simulink model "quantis_filter_1"  (Simulink 7.8)
settings: Solver=FixedStepDiscrete  StartTime=0.0  StopTime=1  RelTol=1e-3
values from neighbouring files (symbols this model uses):
  fs = 16000    [G722_1.m]    (also in TP_fdesign1.m = 0.215; adaptiv_2.m = 1000; adaptiv_3.m = 1000; adaptiv_4.m = 1000)
undefined symbols (not defined in the file or in its folder): dfilt, frs
libraries: dsparch4 x1, dspsrcs4 x1
settings Model: Creator=svenhoffmann  LastModifiedBy=josef  ExtModeAutoUpdateStatusClock=off
settings OptimizationCC: InlineInvariantSignals=on  InitFltsAndDblsToZero=on
settings DebuggingCC: SaveWithParameterizedLinksMsg=none  SignalResolutionControl=TryResolveAllWithWarning  MultiTaskDSMMsg=warning  MultiTaskCondExecSysMsg=none  FcnCallInpInsideContextMsg=Use local settings  StrictBusMsg=None
settings RTWCC: IncludeERTFirstTime=on
settings GRTTargetCC: TargetFcnLib=ansi_tfl_tmw.mat

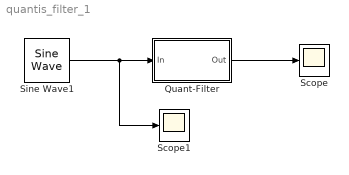
== system quantis_filter_1 ==
  Quant-Filter : Subsystem  Tag=BlockMethodSubSystem
  Scope : Scope
  Scope1 : Scope
  Sine Wave1 : dspsrcs4/Sine Wave  Amplitude=0.95  Frequency=fs/round(1/frs)  Phase=0  SampleMode=Discrete  OutComplex=Real  CompMethod=Table lookup  TableSize=Speed  SampleTime=1/fs  SamplesPerFrame=1  ResetState=Restart at time zero  dataType=User-defined  wordLen=16  udDataType=sfix(16)  fracBitsMode=User-defined  numFracBits=15  OutDataTypeStr=fixdt(1,16)  LastOutDataTypeStr=fixdt(1,16)
  wires:
  Sine Wave1/1 -> Quant-Filter/1(In), Scope1/1
  Quant-Filter/1(Out) -> Scope/1

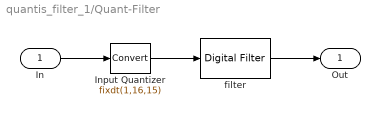
== system quantis_filter_1/Quant-Filter ==
  In : Inport
  Input Quantizer : DataTypeConversion  OutDataTypeStr=fixdt(1,16,15)  RndMeth=Round  SaturateOnIntegerOverflow=on
  filter : dsparch4/Digital Filter  TypePopup=IIR (poles & zeros)  IIRFiltStruct=Direct form II  AllPoleFiltStruct=Direct form  FIRFiltStruct=Direct form  CoeffSource=Specify via dialog  NumCoeffs=[0.000288582897651351 -0.00033839318745116 -0.000390339936011391 -0.000259639046498942 7.38443078093614e-05 0.000357868370809173 0.000300939938371918 -0.000105129054930465 -0.00050182175147418 -0.000461335623672789 7.11317455494947e-05 0.000639924106940051 0.000655538279003823 -8.41836808940086e-06 -0.000791306426059373 -0.000901062859792003 -0.000100245580998996 0.000946038863637751 0.00120070496164748 0.000266513423161963 -0.00109528806843289 -0.00155788027039267 -0.000504175926187551 0.0012271638548347 0.00197432303656502 0.000828029512424704 -0.00132731841121327 -0.00245007010985775 -0.00125334653945962 0.00137873110724473 0.00298262555164426 0.00179638152844382 -0.00136038330873108 -0.00356731415934766 -0.0024752313224474 0.00124855058800306 0.00419864437922346 0.00330857950612985 -0.00101484760130196 -0.00486584907866968 -0.00431926877262247 0.000626112664150373 0.00555922195206759 0.00553337686591329 -4.06558700779738e-05 -0.00626541757131323 -0.00698518729854155 -0.000793203461600921 0.0069706742258114 0.00872392161471349 0.00194621229973601 -0.00765928347665411 -0.0108228080449625 -0.00351974772730628 0.00831542716470059 0.013400989063819 0.00567168379746354 -0.00892343070006198 -0.0166661145296759 -0.00867205472801053 0.00946779586510596 0.0210119633125462 0.0130342493783314 -0.0099347473329221 -0.0272758084634068 -0.0198850138076668 0.0103117218369764 0.0375727529685634 0.0322854051395793 -0.0105884468313137 -0.0591349841236665 -0.0624946230301509 0.0107577655260804 0.142692161023549 0.269992639691952 0.322518460142645 0.269992639691952 0.142692161023549 0.0107577655260804 -0.0624946230301509 -0.0591349841236665 -0.0105884468313137 0.0322854051395793 0.0375727529685634 0.0103117218369764 -0.0198850138076668 -0.0272758084634068 -0.0099347473329221 0.0130342493783314 0.0210119633125462 0.00946779586510596 -0.00867205472801053 -0.0166661145296759 -0.00892343070006198 0.00567168379746354 0.013400989063819 0.00831542716470059 -0.00351974772730628 -0.0108228080449625 -0.00765928347665411 0.00194621229973601 0.00872392161471349 0.0069706742258114 -0.000793203461600921 -0.00698518729854155 -0.00626541757131323 -4.06558700779738e-05 0.00553337686591329 0.00555922195206759 0.000626112664150373 -0.00431926877262247 -0.00486584907866968 -0.00101484760130196 0.00330857950612985 0.00419864437922346 0.00124855058800306 -0.0024752313224474 -0.00356731415934766 -0.00136038330873108 0.00179638152844382 0.00298262555164426 0.00137873110724473 -0.00125334653945962 -0.00245007010985775 -0.00132731841121327 0.000828029512424704 0.00197432303656502 0.0012271638548347 -0.000504175926187551 -0.00155788027039267 -0.00109528806843289 0.000266513423161963 0.00120070496164748 0.000946038863637751 -0.000100245580998996 -0.000901062859792003 -0.000791306426059373 -8.41836808940086e-06 0.000655538279003823 0.000639924106940051 7.11317455494947e-05 -0.000461335623672789 -0.00050182175147418 -0.000105129054930465 0.000300939938371918 0.000357868370809173 7.38443078093614e-05 -0.000259639046498942 -0.000390339936011391 -0.00033839318745116 0.000288582897651351]  DenCoeffs=1  BiQuadCoeffs=[1 0.3 0.4 1 0.1 0.2]  LatticeCoeffs=[0.2 0.4]  denIgnore=on  FiltPerSampPopup=One filter per frame  IC=0  ICnum=0  ICden=0  firstCoeffMode=Binary point scaling  firstCoeffWordLength=16  firstCoeffFracLength=15  outputMode=Binary point scaling  outputWordLength=16  outputFracLength=6  accumMode=Binary point scaling  accumWordLength=40  accumFracLength=30  prodOutputMode=Binary point scaling  prodOutputWordLength=32  prodOutputFracLength=30  memoryMode=Binary point scaling  memoryWordLength=16  memoryFracLength=15  roundingMode=Round  overflowMode=off  ScaleValues=1  scaleValueFracLength=14  stageInFracLength=15  stageOutFracLength=15  FilterSource=Specify via dialog  dfiltObjectName=dfilt.dffir([1 2 1])  InputProcessing=Columns as channels (frame based)
  Out : Outport
  wires:
  In/1 -> Input Quantizer/1
  Input Quantizer/1 -> filter/1
  filter/1 -> Out/1
